simulink model "stateObserver"  (R2018a)
settings: Solver=VariableStepAuto  StartTime=0.0  StopTime=50  RelTol=1e-3
values from neighbouring files (symbols this model uses):
  A = [-1 1;1 -2]    [stateObserverScript.m]    (also in trackingControlScript.m = [-0.01 0;0 -0.02])
  B = [1;1]    [stateObserverScript.m]    (also in trackingControlScript.m = [0.01 0;-0.03 0.04])
  C = eye(2)    [stateObserverScript.m]    (also in trackingControlScript.m = [C1;C2])
  D = [0;0]    [stateObserverScript.m]
  H = H'    [stateObserverScript.m]    (also in trackingControlScript.m = [ zeros(2,2);eye(2,2)])
libraries: simulink x1
settings Model: Creator=Haydar  LastModifiedBy=Haydar

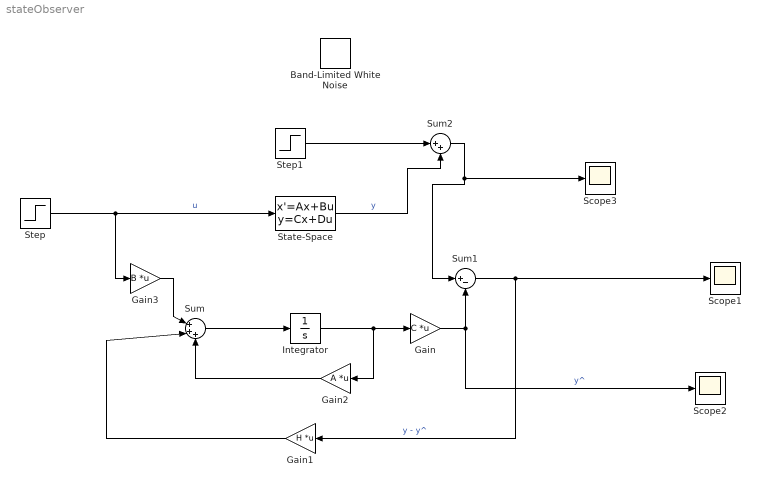
== system stateObserver ==
  Band-Limited White Noise : simulink/Sources/Band-Limited White Noise  Cov=[0.10]  Ts=0.1  seed=[23341]
  Gain : Gain  Gain=C  Multiplication=Matrix(K*u)
  Gain1 : Gain  Gain=H  Multiplication=Matrix(K*u)
  Gain2 : Gain  Gain=A  Multiplication=Matrix(K*u)
  Gain3 : Gain  Gain=B  Multiplication=Matrix(K*u)
  Integrator : Integrator
  Scope1 : Scope
  Scope2 : Scope
  Scope3 : Scope
  State-Space : StateSpace  A=A  B=B  C=C  D=D  InitialCondition=[1 1]'
  Step : Step  Time=0  SampleTime=0
  Step1 : Step  Time=10  After=[0.5;0]  SampleTime=0  VectorParams1D=off
  Sum : Sum  Inputs=|+++
  Sum1 : Sum  Inputs=|+-
  Sum2 : Sum  Inputs=|++
  wires:
  Step/1 -> State-Space/1, Gain3/1  "u"
  Gain3/1 -> Sum/1
  Sum/1 -> Integrator/1
  Integrator/1 -> Gain2/1, Gain/1
  Gain2/1 -> Sum/3
  Gain/1 -> Scope2/1, Sum1/2  "y^"
  Sum1/1 -> Scope1/1, Gain1/1  "y - y^"
  Gain1/1 -> Sum/2
  Step1/1 -> Sum2/1
  State-Space/1 -> Sum2/2  "y"
  Sum2/1 -> Scope3/1, Sum1/1
